simulink model "P413_4_model02"  (R2021a)
settings: Solver=VariableStepAuto  StartTime=0.0  StopTime=tspan(end)  RelTol=1e-3
values from neighbouring files (symbols this model uses):
  Tmax = 296    [P413_4_lc.m]
  Tstart = 285.5    [P413_4_lc.m]
libraries: HORTISIM x6
settings Model: Creator=djoroya  LastModifiedBy=djoroya

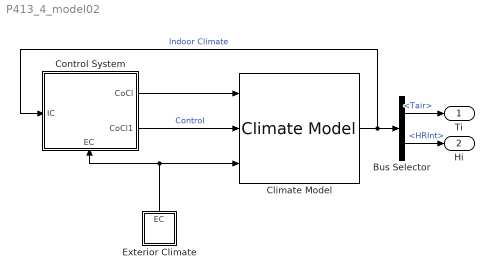
== system P413_4_model02 ==
  Bus Selector : BusSelector  OutputSignals=Temp.Tair,Gas.HRInt
  Climate Model : HORTISIM/Climate/Models/Climate Model  params=p_ic  x0=x0_ic
      settings: SourceProductName=Horti Simulator
  Control System : Subsystem
      settings: PortSchema="{\"entries\":[{\"content\":{\"sides\":[{\"content\":{\"connectorIds\":[\"In1\"]},\"type\":\"ConnectorPlacement.EquallySpacedRectSide\",\"uuid\":\"7d0146e2-a53b-49ab-a7f4-04cd7ef00b9a\"},{\"content\":{\"connectorIds\":[\"Out1\",\"Out2\"],\"side\":\"RIGHT\"},\"type\":\"ConnectorPlacement.EquallySpacedRectSide\",\"uuid\":\"fee587e2-4b5c-4140-8904-07609d427593\"},{\"content\":{\"connectorIds\":[],\"side\":\"TOP\"},\"type\":\"ConnectorPlacement.EquallySpacedRectSide\",\"uuid\":\"52e767bc-1595-40ac-996f-44c9eedd0a08\"},{\"content\":{\"connectorIds\":[\"In2\"],\"side\":\"BOTTOM\"},\"type\":\"ConnectorPlacement.EquallySpacedRectSide\",\"uuid\":\"c629db5c-cfe6-4bd1-aeb9-7fba46dde396\"}]},\"type\":\"ConnectorPlacement.EquallySpacedConnector\",\"uuid\":\"268fde01-3c08-4d62-bfbb-fc94284c5cdd\"}],\"packageUris\":[\"http://schema.mathworks.com/mf0/Connector/R2020b\"],\"version\":\"1.0\"}"
  Exterior Climate : Subsystem
  Ti : Outport
  Hi : Outport  Port=2
  wires:
  Climate Model/1 -> Control System/1(IC), Bus Selector/1  "Indoor Climate"
  Exterior Climate/1(EC) -> Control System/2(EC), Climate Model/3
  Bus Selector/1 -> Ti/1  "<Tair>"
  Bus Selector/2 -> Hi/1  "<HRInt>"
  Control System/1(CoCl) -> Climate Model/1
  Control System/2(CoCl1) -> Climate Model/2  "Control"

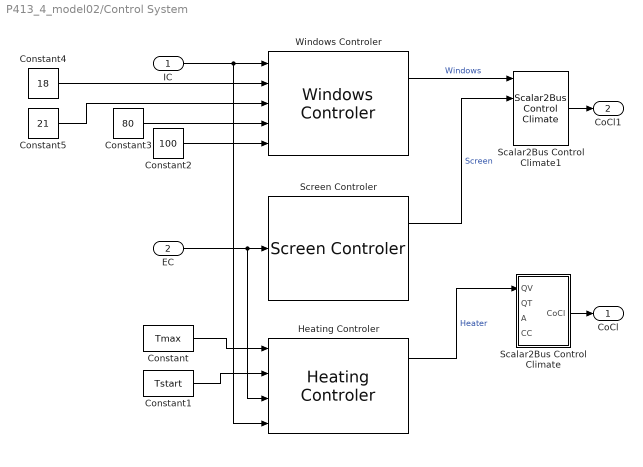
== system P413_4_model02/Control System ==
  IC : Inport
  EC : Inport  Port=2
  Constant : Constant  Value=Tmax
  Constant1 : Constant  Value=Tstart
  Constant2 : Constant  Value=100
  Constant3 : Constant  Value=80
  Constant4 : Constant  Value=18
  Constant5 : Constant  Value=21
  Heating Controler : HORTISIM/Climate/Controls/Heating Controler  params=HP  x0=x0_H
      settings: SourceProductName=Horti Simulator
  Scalar2Bus Control Climate : Subsystem
  Scalar2Bus Control Climate1 : HORTISIM/Other  Functions/Scalar2Bus  Control Climate  SystemSampleTime=-1  VariantActivationTime=update diagram  Latency=0  AutoFrameSizeCalculation=off
      settings: SourceProductName=Horti Simulator
  Screen Controler : HORTISIM/Climate/Controls/Screen Controler  params=scr_p
      settings: SourceProductName=Horti Simulator
  Windows Controler : HORTISIM/Climate/Controls/Windows Controler  params=win_p
      settings: SourceProductName=Horti Simulator
  CoCl : Outport
  CoCl1 : Outport  Port=2
  wires:
  EC/1 -> Heating Controler/3, Screen Controler/1
  Scalar2Bus Control Climate/1(CoCl) -> CoCl/1
  Heating Controler/1 -> Scalar2Bus Control Climate/1(QV)  "Heater"
  Constant1/1 -> Heating Controler/2
  Constant/1 -> Heating Controler/1
  Windows Controler/1 -> Scalar2Bus Control Climate1/1  "Windows"
  Scalar2Bus Control Climate1/1 -> CoCl1/1
  Screen Controler/1 -> Scalar2Bus Control Climate1/2  "Screen"
  IC/1 -> Heating Controler/4, Windows Controler/1
  Constant2/1 -> Windows Controler/5
  Constant3/1 -> Windows Controler/4
  Constant4/1 -> Windows Controler/2
  Constant5/1 -> Windows Controler/3

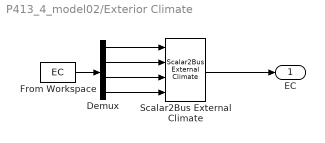
== system P413_4_model02/Exterior Climate ==
  Demux : Demux
  From Workspace : FromWorkspace  VariableName=EC
  Scalar2Bus External Climate : HORTISIM/Other  Functions/Scalar2Bus External Climate  SystemSampleTime=-1  VariantActivationTime=update diagram  Latency=0  AutoFrameSizeCalculation=off
      settings: SourceProductName=Horti Simulator
  EC : Outport
  wires:
  Demux/3 -> Scalar2Bus External Climate/3
  Demux/2 -> Scalar2Bus External Climate/2
  Scalar2Bus External Climate/1 -> EC/1
  Demux/1 -> Scalar2Bus External Climate/1
  Demux/4 -> Scalar2Bus External Climate/4
  From Workspace/1 -> Demux/1

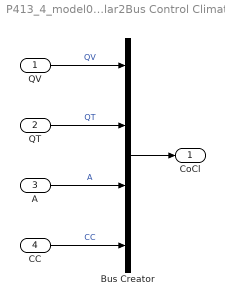
== system P413_4_model02/Control System/Scalar2Bus Control Climate ==
  QV : Inport
  QT : Inport  Port=2
  A : Inport  Port=3
  CC : Inport  Port=4
  Bus Creator : BusCreator  Inputs=4
  CoCl : Outport
  wires:
  A/1 -> Bus Creator/3  "A"
  CC/1 -> Bus Creator/4  "CC"
  QV/1 -> Bus Creator/1  "QV"
  Bus Creator/1 -> CoCl/1
  QT/1 -> Bus Creator/2  "QT"
